simulink model "LQR_Control_model"  (R2023a)
settings: Solver=VariableStepAuto  StartTime=0.0  StopTime=2  RelTol=1e-3
undefined symbols (not defined in the file): A, B, C, D, E, K3
settings Model: Creator=z'k'x  LastModifiedBy=z'k'x

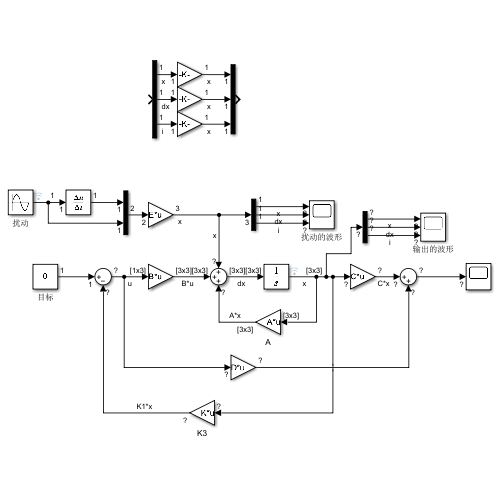
[thumbnail: Simulink's stored preview of the top-level diagram]
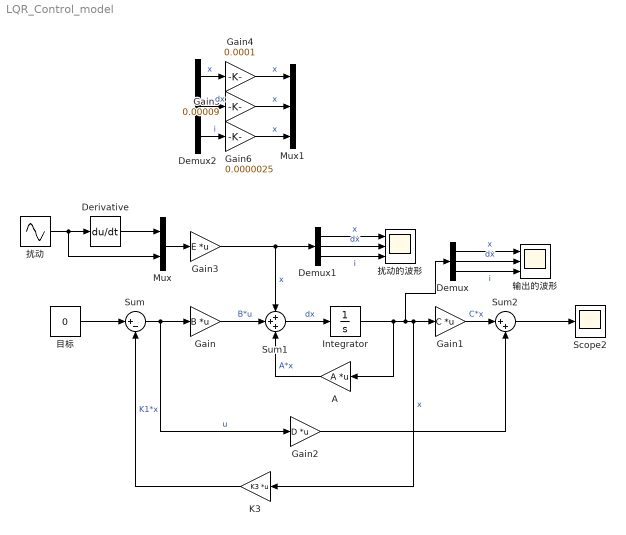
== system LQR_Control_model ==
  A : Gain  Gain=A  Multiplication=Matrix(K*u)
  Demux : Demux  Outputs=3
  Demux1 : Demux  Outputs=3
  Demux2 : Demux  Outputs=3
  Derivative : Derivative
  Gain : Gain  Gain=B  Multiplication=Matrix(K*u)
  Gain1 : Gain  Gain=C  Multiplication=Matrix(K*u)
  Gain2 : Gain  Gain=D  Multiplication=Matrix(K*u)
  Gain3 : Gain  Gain=E  Multiplication=Matrix(K*u)
  Gain4 : Gain  Gain=0.0001
  Gain5 : Gain  Gain=0.00009
  Gain6 : Gain  Gain=0.0000025
  Integrator : Integrator
  K3 : Gain  Gain=K3  Multiplication=Matrix(K*u)
  Mux : Mux  Inputs=2
  Mux1 : Mux  Inputs=3
  Scope2 : Scope
  Sum : Sum  Inputs=|+-
  Sum1 : Sum  Inputs=+++
  Sum2 : Sum  Inputs=|++
  扰动 : Sin  Frequency=17.38*2*pi  SampleTime=0
  扰动的波形 : Scope  NumInputPorts=3
  目标 : Constant  Value=0
  输出的波形 : Scope  NumInputPorts=3
  wires:
  Sum/1 -> Gain2/1, Gain/1  "u"
  Gain/1 -> Sum1/2  "B*u"
  Sum1/1 -> Integrator/1  "dx"
  Integrator/1 -> A/1, Demux/1, K3/1, Gain1/1  "x"
  Gain1/1 -> Sum2/1  "C*x"
  A/1 -> Sum1/3  "A*x"
  K3/1 -> Sum/2  "K1*x"
  Gain2/1 -> Sum2/2
  Derivative/1 -> Mux/1
  扰动/1 -> Mux/2, Derivative/1
  Mux/1 -> Gain3/1
  Demux/1 -> 输出的波形/1  "x"
  Sum2/1 -> Scope2/1
  Demux/2 -> 输出的波形/2  "dx"
  Demux/3 -> 输出的波形/3  "i"
  Demux1/3 -> 扰动的波形/3  "i"
  Demux1/2 -> 扰动的波形/2  "dx"
  Gain3/1 -> Demux1/1, Sum1/1  "x"
  Demux1/1 -> 扰动的波形/1  "x"
  Gain6/1 -> Mux1/3  "x"
  Demux2/3 -> Gain6/1  "i"
  Gain4/1 -> Mux1/1  "x"
  Gain5/1 -> Mux1/2  "x"
  Demux2/2 -> Gain5/1  "dx"
  Demux2/1 -> Gain4/1  "x"
  目标/1 -> Sum/1
